simulink model "lqrinputquaternion"  (R2014a)
settings: Solver=ode45  StartTime=0.0  StopTime=10.0  RelTol=1e-3
undefined symbols (not defined in the file): DiscIntNeverNeededParam, k
libraries: aerolibutil x2, aerolibtransform2 x2
settings Model: Creator=aman  LastModifiedBy=aman

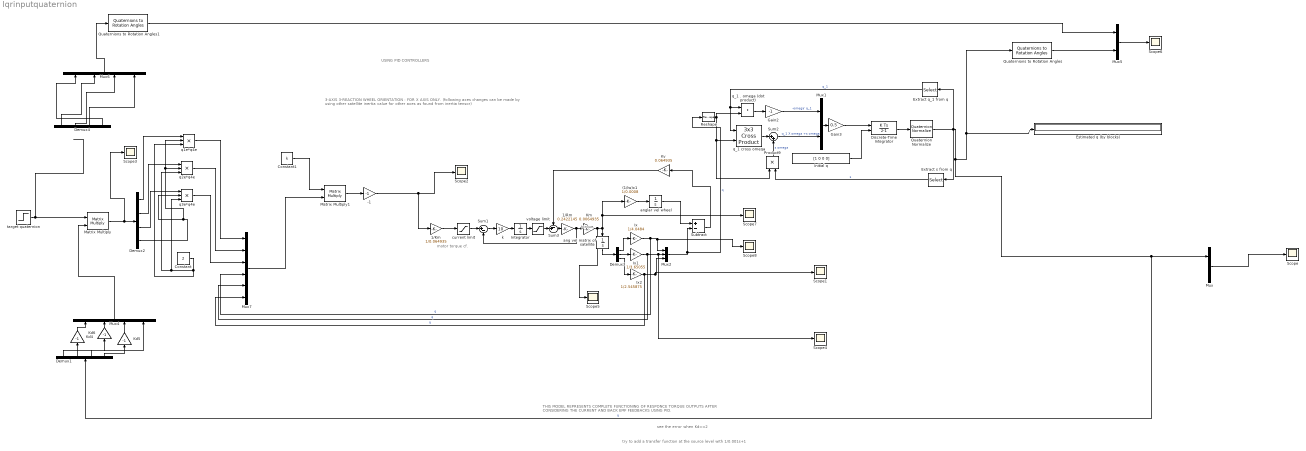
== system lqrinputquaternion ==
  note: try to add a transfer function at the source level with 1/0.001s+1
  note: see the error when Kd>=2
  note: USING PID CONTROLLERS
  note: 3-AXIS 3-REACTION WHEEL ORIENTATION : FOR X AXIS ONLY.
      | (following axes changes can be made by using other satellite inertia value for other axes as found from inertia tensor)
  note: torque
  note: THIS MODEL REPRESENTS COMPLETE FUNCTIONING OF RESPONCE TORQUE OUTPUTS AFTER CONSIDERING THE CURRENT AND BACK EMF FEEDBACKS USING PID.
  note: motor
      | torque
      | cf.
  (1/Iw)x1 : Gain  Gain=1/0.0008
  -1 : Gain  Gain=-1
  1/Km : Gain  Gain=1/0.064935
  1/Rm : Gain  Gain=0.2422145
  Constant : Constant  Value=2
  Constant1 : Constant  Value=k
  Demux1 : Demux
  Demux2 : Demux
  Demux3 : Demux  Outputs=3
  Demux4 : Demux
  Discrete-Time Integrator : DiscreteIntegrator  InitialConditionSource=external  SampleTime=0.1  ICPrevOutput=DiscIntNeverNeededParam  ICPrevScaledInput=DiscIntNeverNeededParam
  Estimated q (by blocks) : Display
  Extract q_1 from q : Selector  InputPortWidth=4  Indices=[2:4]
  Extract s from q : Selector  InputPortWidth=4
  Gain2 : Gain  Gain=-1  SaturateOnIntegerOverflow=on  OutDataTypeStr=Inherit: Same as input  ParamDataTypeStr=Inherit: Same as input
  Gain3 : Gain  Gain=0.5  SaturateOnIntegerOverflow=on  OutDataTypeStr=Inherit: Same as input  ParamDataTypeStr=Inherit: Same as input
  "Initial q " : Constant  Value=[1 0 0 0]  VectorParams1D=off
  Integrator : Integrator
  Ix : Gain  Gain=1/4.0484
  Ix1 : Gain  Gain=1/3.65055
  Ix2 : Gain  Gain=1/2.545875
  Kd4 : Gain  Gain=-1
  Kd5 : Gain  Gain=-1
  Kd6 : Gain  Gain=-1
  Km : Gain  Gain=0.0064935
  Kv : Gain  Gain=0.064935
  Matrix Multiply : Product  Multiplication=Matrix(*)
  Matrix Multiply1 : Product  Multiplication=Matrix(*)
  Mux : Mux  Inputs=2
  Mux1 : Mux  Inputs=2
  Mux2 : Mux  Inputs=3
  Mux4 : Mux
  Mux5 : Mux  Inputs=2
  Mux6 : Mux
  Mux7 : Mux  Inputs=6
  Product9 : Product  Inputs=**  SaturateOnIntegerOverflow=on  InputSameDT=on  OutDataTypeStr=Inherit: Same as first input
  Quaternion Normalize : aerolibutil/Quaternion Normalize
  Quaternions to Rotation Angles : aerolibtransform2/Quaternions to Rotation Angles  rotationOrder=XYZ
  Quaternions to Rotation Angles1 : aerolibtransform2/Quaternions to Rotation Angles  rotationOrder=XYZ
  Reshape : Reshape  OutputDimensionality=Row vector (2-D)
  Scope{,1..8} (9 alike) : Scope
      Scope settings: TimeRange=600  YMin=-1  YMax=1  SaveName=ScopeData2
      Scope3 settings: SaveName=ScopeData3
      Scope4 settings: SaveName=ScopeData4
      Scope5 settings: SaveName=ScopeData5
      Scope6 settings: SaveName=ScopeData6
      Scope7 settings: SaveName=ScopeData7
      Scope8 settings: SaveName=ScopeData8
  Subtract : Sum  Inputs=+-
  Sum1 : Sum  Inputs=|+-
  Sum2 : Sum  Inputs=|++  SaturateOnIntegerOverflow=on
  Sum3 : Sum  Inputs=-+|
  ang vel matrix of satellite : Integrator
  anglar vel wheel : Integrator
  current limit : Saturate  UpperLimit=0.8  LowerLimit=-0.8
  k : Gain  Gain=10
  q1e*q4e : Product  Inputs=3
  q2e*q4e : Product  Inputs=3
  q3e*q4e : Product  Inputs=3
  q_1 . omega (dot product) : DotProduct  InputSameDT=on  OutDataTypeStr=Inherit: Inherit via internal rule
  q_1 cross omeqa : aerolibutil/3x3 Cross Product
  target quaternion : Step  Before=[1,0,0,0;0,1,0,0;0,0,1,0;0,0,0,1]  After=[0.9723,0.1452,-0.1114,0.1452;-0.1452,0.9723,0.1452,0.1114;0.1114,-0.1452,0.9723,0.1452;-0.1452,-0.1114,-0.1452,0.9723]  SampleTime=0
  voltage limit : Saturate  UpperLimit=35  LowerLimit=-35
  wires:
  1/Km/1 -> current limit/1
  k/1 -> Integrator/1
  Integrator/1 -> voltage limit/1
  1/Rm/1 -> Sum1/2, Km/1
  current limit/1 -> Sum1/1
  Sum1/1 -> k/1
  Sum3/1 -> 1/Rm/1
  voltage limit/1 -> Sum3/2
  Demux2/4 -> q2e*q4e/2, q1e*q4e/2, q3e*q4e/2
  (1/Iw)x1/1 -> anglar vel wheel/1
  anglar vel wheel/1 -> Subtract/1
  Subtract/1 -> Kv/1
  Kv/1 -> Sum3/1
  Mux/1 -> Scope/1
  Matrix Multiply/1 -> Scope3/1, Demux2/1
  Demux3/2 -> Ix1/1
  Demux3/3 -> Ix2/1
  Demux3/1 -> Ix/1
  Km/1 -> Scope5/1, ang vel matrix of satellite/1, Scope7/1, (1/Iw)x1/1
  Extract s from q/1 -> Product9/2  "s"
  Gain3/1 -> Discrete-Time Integrator/1
  Mux1/1 -> Gain3/1
  Gain2/1 -> Mux1/1  "-omega' q_1"
  Sum2/1 -> Mux1/2  "q_1 X omega +s omega"
  q_1 . omega (dot product)/1 -> Gain2/1
  Quaternion Normalize/1 -> Extract s from q/1, Extract q_1 from q/1, Demux1/1, Mux/1, Quaternions to Rotation Angles/1, Estimated q (by blocks)/1  "q"
  Discrete-Time Integrator/1 -> Quaternion Normalize/1
  "Initial q "/1 -> Discrete-Time Integrator/2
  q_1 cross omeqa/1 -> Sum2/1
  Product9/1 -> Sum2/2  "s omega"
  Extract q_1 from q/1 -> q_1 cross omeqa/1, q_1 . omega (dot product)/1  "q_1"
  Reshape/1 -> q_1 . omega (dot product)/2, q_1 cross omeqa/2, Product9/1
  Demux1/2 -> Kd4/1
  Demux1/3 -> Kd6/1
  Demux1/4 -> Kd5/1
  Demux1/1 -> Mux4/4
  Quaternions to Rotation Angles/1 -> Mux5/2
  target quaternion/1 -> Matrix Multiply/1
  Quaternions to Rotation Angles1/1 -> Mux5/1
  Mux5/1 -> Scope6/1
  Demux4/2 -> Mux6/3
  Demux4/3 -> Mux6/4
  Demux4/4 -> Mux6/1
  Demux4/1 -> Mux6/2
  Mux6/1 -> Quaternions to Rotation Angles1/1
  Kd4/1 -> Mux4/1
  Kd6/1 -> Mux4/2
  Kd5/1 -> Mux4/3
  Mux4/1 -> Matrix Multiply/2
  Mux2/1 -> Reshape/1, Subtract/2  "q"
  ang vel matrix of satellite/1 -> Demux3/1
  Ix2/1 -> Mux7/6, Scope1/1, Mux2/3  "q"
  Ix1/1 -> Mux7/5, Scope4/1, Mux2/2  "q"
  Ix/1 -> Mux7/4, Scope8/1, Mux2/1  "q"
  -1/1 -> 1/Km/1, Scope2/1
  Demux2/1 -> q1e*q4e/1
  Demux2/2 -> q2e*q4e/1
  Demux2/3 -> q3e*q4e/1
  Constant/1 -> q1e*q4e/3, q2e*q4e/3, q3e*q4e/3
  q1e*q4e/1 -> Mux7/1
  q2e*q4e/1 -> Mux7/2
  q3e*q4e/1 -> Mux7/3
  Mux7/1 -> Matrix Multiply1/2
  Matrix Multiply1/1 -> -1/1
  Constant1/1 -> Matrix Multiply1/1
